simulink model "SIMWORKING"  (R2023b)
settings: Solver=VariableStepAuto  StartTime=0.0  StopTime=inf  RelTol=1e-3
undefined symbols (not defined in the file): deg, fractalcoef, IC, K, m, O, rad, s
libraries: aerolibconvert2 x7, sensorinslib x3, aerolibanimutils x3, simulink x3, aerolibnav x3, mspsensorlib x1, aerolibatmos2 x1, vrlib x1, aerolibasang x1, aerolibsim3d x1, sim3dlib x1
settings Model: Creator=kerley0  LastModifiedBy=pizza

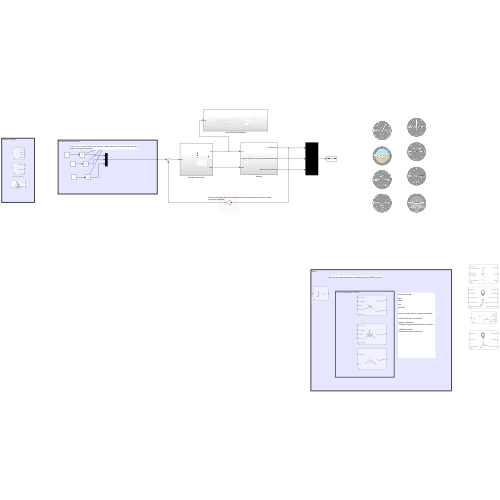
[thumbnail: Simulink's stored preview of the top-level diagram]
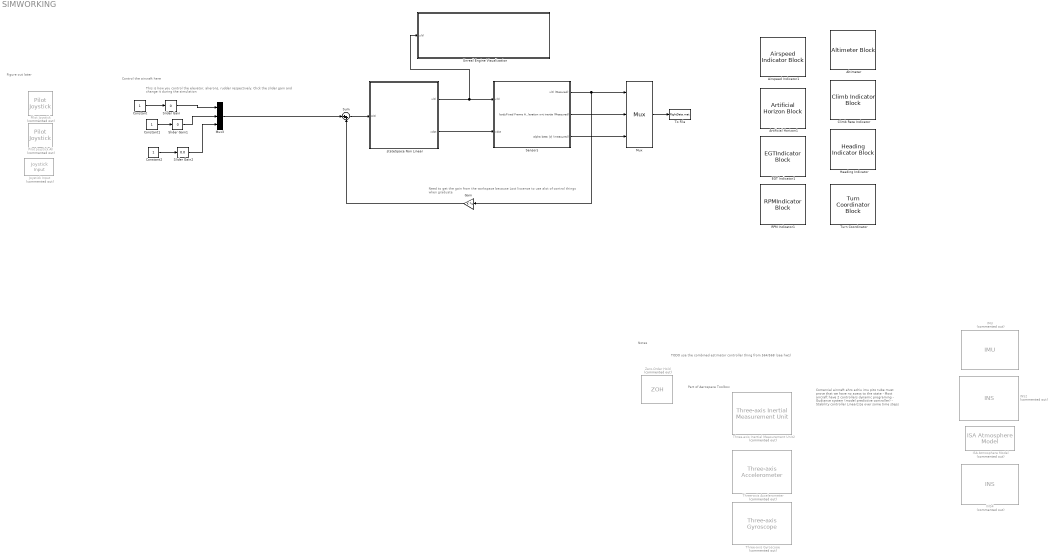
== system SIMWORKING ==
  note: Need to get the gain from the workspace because Lost liscence to use alot of control things when graduate
  note: TODO use the combined estimator controller thing from 564/568 (see hw1)
  note: Figure out later
  note: Notes
  note: Part of Aerospace Toolbox
  note: Comercial aircraft
      |
      | ahrs
      | adriu
      |
      | imu
      | pito tube
      |
      |
      | must prove that we have no acess to the state
      |
      | - Most aircraft have 2 controllers
      |
      | dynamic programing
      | - Gudiance system (model predictive controller)
      |
      | - Stability controller
      | Linearzize over some time steps
  note: Control the aircraft here
  note: This is how you control the elevator, alierons, rudder respectively. Click the slider gain and change it during the simulation
  Airspeed Indicator1 : AirspeedIndicatorBlock
  Altimeter : AltimeterBlock
  Artificial Horizon1 : ArtificialHorizonBlock
  Climb Rate Indicator : ClimbIndicatorBlock
  Constant : Constant
  Constant1 : Constant
  Constant2 : Constant
  EGT Indicator1 : EGTIndicatorBlock
  Gain : Gain  Gain=K  Multiplication=Matrix(K*u)
  Heading Indicator : HeadingIndicatorBlock
  IMU : mspsensorlib/IMU  Commented=on  DispRefFrame=NED  TemperaturePort=off  Temperature=25  MagneticFieldPort=off  MagneticFieldNED=[ 27.5550, -2.4169, -16.0849 ]  MagneticFieldENU=[ -2.4169, 27.5550, 16.0849 ]  SeedDouble=67  SimulateUsing=Interpreted execution  AccelParamsMeasurementRange=Inf  AccelParamsResolution=0  AccelParamsConstantBias=[ 0, 0, 0 ]  AccelParamsAxesMisalignment=[ 100, 0, 0; 0, 100, 0; 0, 0, 100 ]  AccelParamsNoiseDensity=[ 0, 0, 0 ]  AccelParamsBiasInstability=[ 0, 0, 0 ]  AccelParamsBiasInstabilityNumerator=fractalcoef().Numerator  AccelParamsBiasInstabilityDenominator=fractalcoef().Denominator  AccelParamsRandomWalk=[ 0, 0, 0 ]  AccelParamsNoiseType=double-sided  AccelParamsTemperatureBias=[ 0, 0, 0 ]  AccelParamsTemperatureScaleFactor=[ 0, 0, 0 ]  GyroParamsMeasurementRange=Inf  GyroParamsResolution=0  GyroParamsConstantBias=[ 0, 0, 0 ]  GyroParamsAxesMisalignment=[ 100, 0, 0; 0, 100, 0; 0, 0, 100 ]  GyroParamsAccelerationBias=[ 0, 0, 0 ]  GyroParamsNoiseDensity=[ 0, 0, 0 ]  GyroParamsBiasInstability=[ 0, 0, 0 ]  GyroParamsBiasInstabilityNumerator=fractalcoef().Numerator  GyroParamsBiasInstabilityDenominator=fractalcoef().Denominator  GyroParamsRandomWalk=[ 0, 0, 0 ]  GyroParamsNoiseType=double-sided  GyroParamsTemperatureBias=[ 0, 0, 0 ]  GyroParamsTemperatureScaleFactor=[ 0, 0, 0 ]  MagParamsMeasurementRange=Inf  MagParamsResolution=0  MagParamsConstantBias=[ 0, 0, 0 ]  MagParamsAxesMisalignment=[ 100, 0, 0; 0, 100, 0; 0, 0, 100 ]  MagParamsNoiseDensity=[ 0, 0, 0 ]  MagParamsBiasInstability=[ 0, 0, 0 ]  MagParamsBiasInstabilityNumerator=fractalcoef().Numerator  MagParamsBiasInstabilityDenominator=fractalcoef().Denominator  MagParamsRandomWalk=[ 0, 0, 0 ]  MagParamsNoiseType=double-sided  MagParamsTemperatureBias=[ 0, 0, 0 ]  MagParamsTemperatureScaleFactor=[ 0, 0, 0 ]
  INS2 : sensorinslib/INS  Commented=on  MountingLocation=[0 0 0]  RollAccuracy=0.2  PitchAccuracy=0.2  YawAccuracy=1  PositionAccuracy=1  VelocityAccuracy=0.05  UseAccelAndAngVel=on  AccelerationAccuracy=0  AngularVelocityAccuracy=0  TimeInput=off  PositionErrorFactor=[0 0 0]  SeedDouble=67  SimulateUsing=Interpreted execution
      settings: LibrarySourceBlock=uavsimlib/INS
  INS4 : sensorinslib/INS  Commented=on  MountingLocation=[0 0 0]  RollAccuracy=0.2  PitchAccuracy=0.2  YawAccuracy=1  PositionAccuracy=1  VelocityAccuracy=0.05  UseAccelAndAngVel=off  AccelerationAccuracy=0  AngularVelocityAccuracy=0  TimeInput=off  PositionErrorFactor=[0 0 0]  SeedDouble=67  SimulateUsing=Interpreted execution
      settings: LibrarySourceBlock=uavsimlib/INS
  ISA Atmosphere Model : aerolibatmos2/ISA Atmosphere Model  Commented=on  useExtended=off  action=Warning  custom=off  viscosityOut=off  g=9.80665  gamma=1.4  R=287.0531  L=0.0065  h_trop=11000  h_strat=20000  rho0=1.225  P0=101325  T0=288.15  h0=0
  Joystick Input : vrlib/Joystick Input  Commented=on  joyid=1  adjustports=on  forcefeed=off
  Mux : Mux  Inputs=3
  Mux3 : Mux  Inputs=3
  Pilot Joystick : aerolibanimutils/Pilot Joystick  Commented=on  JoystickID=Joystick1  OutputConfiguration=FourAxis  SampleTime=1/30
  Pilot Joystick All : aerolibanimutils/Pilot Joystick  Commented=on  JoystickID=Joystick1  OutputConfiguration=AllOutputs  SampleTime=1/30
      settings: LibrarySourceBlock=aerolibanimutils/Pilot Joystick All
  RPM Indicator1 : RPMIndicatorBlock
  Sensors : Subsystem
  Slider Gain : simulink/Math Operations/Slider Gain  gain=0  low=-0.4363  high=0.4363
  Slider Gain1 : simulink/Math Operations/Slider Gain  gain=0  low=-0.4363  high=0.4363
  Slider Gain2 : simulink/Math Operations/Slider Gain  gain=0.0  low=-0.6  high=0.6
  Sum : Sum  Inputs=|++
  Three-axis Accelerometer : aerolibnav/Three-axis Accelerometer  Commented=on  units=Metric (MKS)  acc=[0 0 0]  gtype=on  dtype_a=on  w_a=190  z_a=0.707  a_sf_cc=[1 0 0; 0 1 0; 0 0 1]  a_bias=[0 0 0]  a_Ts=0  a_rand=on  a_seeds=[23093 23094 23095]  a_pow=[0.001 0.001 0.001]  a_sat="[-inf  -inf  -inf  inf inf inf]"
  Three-axis Gyroscope : aerolibnav/Three-axis Gyroscope  Commented=on  dtype_g=on  w_g=190  z_g=0.707  g_sf_cc=[1 0 0; 0 1 0; 0 0 1]  g_bias=[0 0 0]  g_sen=[0 0 0]  g_Ts=0  g_rand=on  g_seeds=[23093 23094 23095]  g_pow=[0.0001 0.0001 0.0001]  g_sat="[-inf  -inf  -inf  inf inf inf]"
  Three-axis Inertial Measurement Unit2 : aerolibnav/Three-axis Inertial Measurement Unit  Commented=on  units=Metric (MKS)  imu=[0 0 0]  i_Ts=0  dtype_a=on  w_a=190  z_a=0.707  a_sf_cc=[1 0 0; 0 1 0; 0 0 1]  a_bias=[0 0 0]  a_sat="[-inf  -inf  -inf  inf inf inf]"  dtype_g=on  w_g=190  z_g=0.707  g_sf_cc=[1 0 0; 0 1 0; 0 0 1]  g_bias=[0 0 0]  g_sens=[0 0 0]  g_sat="[-inf  -inf  -inf  inf inf inf]"  i_rand=on  i_seeds=[23093 23094 23095 23096 23097 23098]  i_pow=[0.001 0.001 0.001 0.0001 0.0001 0.0001]
  To File : ToFile  Filename=flightData.mat
  Turn Coordinator : TurnCoordinatorBlock
  Unreal Engine Visualization : Subsystem
  Zero-Order Hold : ZeroOrderHold  Commented=on  SampleTime=-1
  stateSpace Non Linear : Subsystem
  wires:
  Slider Gain/1 -> Mux3/1
  Constant/1 -> Slider Gain/1
  Constant1/1 -> Slider Gain1/1
  Constant2/1 -> Slider Gain2/1
  Slider Gain2/1 -> Mux3/3
  Slider Gain1/1 -> Mux3/2
  Mux3/1 -> Sum/1
  stateSpace Non Linear/2(" xdot") -> Sensors/2(xdot)
  stateSpace Non Linear/1(x(t)) -> Sensors/1(x(t)), Unreal Engine Visualization/1(y(t))
  Sensors/3(alpha beta |V| (measured)) -> Mux/3
  Sensors/2(bodyFixed Frame Acceleration wrt inertia (Measured)) -> Mux/2
  Sensors/1(x(t) (Mesured)) -> Gain/1, Mux/1
  Mux/1 -> To File/1
  Sum/1 -> stateSpace Non Linear/1(U(t))
  Gain/1 -> Sum/2

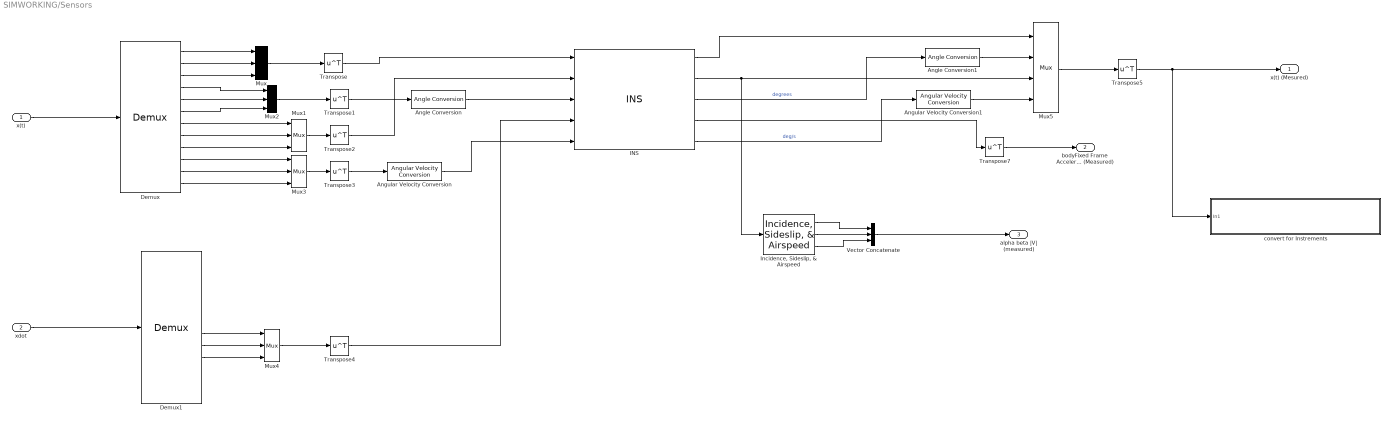
== system SIMWORKING/Sensors ==
  x(t) : Inport
  xdot : Inport  Port=2
  Angle Conversion : aerolibconvert2/Angle Conversion  IU=rad  OU=deg
  Angle Conversion1 : aerolibconvert2/Angle Conversion  IU=deg  OU=rad
  Angular Velocity Conversion : aerolibconvert2/Angular Velocity Conversion  IU=rad/s  OU=deg/s
  Angular Velocity Conversion1 : aerolibconvert2/Angular Velocity Conversion  IU=deg/s  OU=rad/s
  Demux : Demux  Outputs=12
  Demux1 : Demux  Outputs=12
  INS : sensorinslib/INS  MountingLocation=[0 0 0]  RollAccuracy=5  PitchAccuracy=5  YawAccuracy=5  PositionAccuracy=5  VelocityAccuracy=5  UseAccelAndAngVel=on  AccelerationAccuracy=1  AngularVelocityAccuracy=1  TimeInput=off  PositionErrorFactor=[0 0 0]  SeedDouble=67  SimulateUsing=Code generation
      settings: LibrarySourceBlock=mspsensorlib/INS
  "Incidence, Sideslip, & Airspeed" : aerolibasang/Incidence, Sideslip, & Airspeed
  Mux{,1..4} (5 alike) : Mux  Inputs=3
  Mux5 : Mux
  Transpose{,1..5,7} (7 alike) : Math  Operator=transpose
  Vector Concatenate : Concatenate  NumInputs=3
  convert for Instrements : Subsystem
  x(t) (Mesured) : Outport
  bodyFixed Frame Acceleration wrt inertia (Measured) : Outport  Port=2
  alpha beta |V| (measured) : Outport  Port=3
  wires:
  Transpose4/1 -> INS/4
  INS/1 -> Mux5/1
  Transpose1/1 -> Angle Conversion/1
  INS/5 -> Angular Velocity Conversion1/1  "deg/s"
  x(t)/1 -> Demux/1
  INS/3 -> Angle Conversion1/1  "degrees"
  Transpose3/1 -> Angular Velocity Conversion/1
  Demux/1 -> Mux/1
  Demux/2 -> Mux/2
  Demux/3 -> Mux/3
  Mux/1 -> Transpose/1
  Transpose/1 -> INS/1
  Demux/4 -> Mux2/1
  Demux/5 -> Mux2/2
  Demux/6 -> Mux2/3
  Mux2/1 -> Transpose1/1
  Demux/7 -> Mux1/1
  Demux/8 -> Mux1/2
  Demux/9 -> Mux1/3
  Mux1/1 -> Transpose2/1
  Transpose2/1 -> INS/2
  Demux/10 -> Mux3/1
  Demux/11 -> Mux3/2
  Demux/12 -> Mux3/3
  Mux3/1 -> Transpose3/1
  xdot/1 -> Demux1/1
  Demux1/7 -> Mux4/1
  Demux1/8 -> Mux4/2
  Demux1/9 -> Mux4/3
  Mux4/1 -> Transpose4/1
  Mux5/1 -> Transpose5/1
  Transpose5/1 -> convert for Instrements/1(In1), x(t) (Mesured)/1
  Angular Velocity Conversion/1 -> INS/5
  Angle Conversion/1 -> INS/3
  INS/2 -> "Incidence, Sideslip, & Airspeed"/1, Mux5/3
  INS/4 -> Transpose7/1
  Angular Velocity Conversion1/1 -> Mux5/4
  Angle Conversion1/1 -> Mux5/2
  "Incidence, Sideslip, & Airspeed"/1 -> Vector Concatenate/1
  "Incidence, Sideslip, & Airspeed"/2 -> Vector Concatenate/2
  "Incidence, Sideslip, & Airspeed"/3 -> Vector Concatenate/3
  Vector Concatenate/1 -> alpha beta |V| (measured)/1
  Transpose7/1 -> bodyFixed Frame Acceleration wrt inertia (Measured)/1

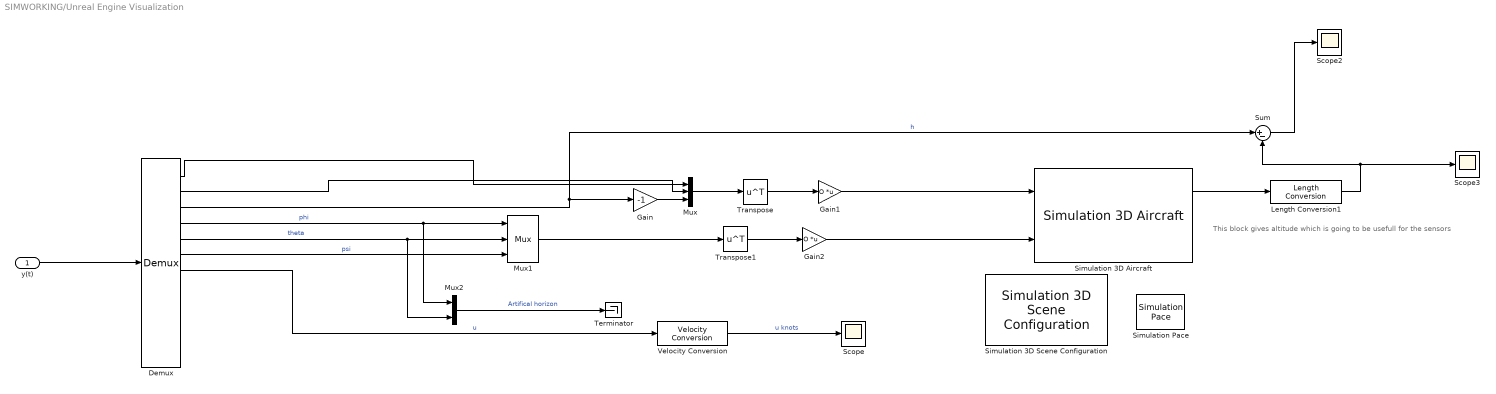
== system SIMWORKING/Unreal Engine Visualization ==
  note: This block gives altitude which is going to be usefull for the sensors
  y(t) : Inport
  Demux : Demux  Outputs=12
  Gain : Gain  Gain=-1
  Gain1 : Gain  Gain=O  Multiplication=Matrix(K*u)
  Gain2 : Gain  Gain=O  Multiplication=Matrix(K*u)
  Length Conversion1 : aerolibconvert2/Length Conversion  IU=m  OU=ft
  Mux : Mux  Inputs=3
  Mux1 : Mux  Inputs=3
  Mux2 : Mux  Inputs=2
  Scope : Scope
  Scope2 : Scope
  Scope3 : Scope
  Simulation 3D Aircraft : aerolibsim3d/Simulation 3D Aircraft  Priority=-1  Mesh=Sky Hogg  MeshPath=/MathWorksAerospaceContent/Vehicles/Aircraft/Custom/Mesh/SK_HL20.SK_HL20  MeshPathAT=/MathWorksAerospaceContent/Vehicles/Aircraft/AirTransport/Mesh/SK_AirTransport.SK_AirTransport  MeshPathGA=/MathWorksAerospaceContent/Vehicles/Aircraft/GeneralAviation/Mesh/SK_GeneralAviation.SK_GeneralAviation  AircraftColor=Red  ActorName=SimulinkVehicle1  Translation=zeros( 11, 3 )  Rotation=zeros( 11, 3 )  IsGHSensorEnabled=on  AreGHRaysVisible=off  IsOutputReshapeEnabled=off  GHRayLength=1524  GHBodyOffset=0.90  GHFrontTireRadius=0.21  GHLeftTireRadius=0.21  GHRightTireRadius=0.21  WoWSensorTolerance=0.05  LightsConfig=Automatic lights  LandingLightIntensity=300000  LandingLightConeAngle=15  CustomLeftLandingLightLocation=[0 0 0]  CustomLeftLandingLightOrientation=[0 0 0]  CustomRightLandingLightLocation=[0 0 0]  CustomRightLandingLightOrientation=[0 0 0]  TaxiLightIntensity=150000  TaxiLightConeAngle=36  CustomTaxiLightLocation=[0 0 0]  CustomTaxiLightOrientation=[0 0 0]  NavLightIntensity=500  PositionLightIntensity=500  StrobeLightIntensity=5000  WingtipStrobePeriod=1.5  WingtipStrobePulseWidth=6  TailStrobePeriod=1.5  TailStrobePulseWidth=6  BeaconLightIntensity=4000  BeaconPeriod=1.5  BeaconPulseWidth=10  SampleTime=-1  ActorType=SimulinkVehicle  ID=1  aMode=0  ActorTag=SimulinkVehicle1
  Simulation 3D Scene Configuration : sim3dlib/Simulation 3D Scene Configuration  Priority=0  ProjectFormat=Default Scenes  SceneDesc=Airport  ProjectName=C:\Program Files\MATLAB\R2023b\toolbox\shared\sim3d_projects\automotive_project_windows\UE\WindowsNoEditor\VehicleSimulation.exe  ScenePath=/Game/Maps/HwStrght  EnableOpenDRIVE=off  vehTagList={'Scene Origin';'SimulinkVehicle1'}  vehTag=SimulinkVehicle1  FreeCameraInitialTranslation=[0, 0, 0]  FreeCameraDefaultInitialTranslation=[-6, 0, 2]  FreeCameraInitialRotation=[0, 0, 0]  FreeCameraDefaultInitialRotation=[0, -15, 0]  OpVisEn=off  Ts=0.01  EnableWindow=on  EnableRemoteAccess=off  EnableWeather=off  SunAltitude=40.0  SunAzimuth=90  clouds=10  wind=1  fog=0  rain=0  EnableGeospatial=off  OriginHeight=200  OriginLatitude=40.744652  OriginLongitude=-73.988864  MapStyle=Aerial  AdditionalAssetIDs=[]  UseAdvancedSunSky=off  SolarTime=11  TimeZone=-5  Day=21  Month=9  Year=2022  UseDaylightSavingTime=on  DSTStartDay=10  DSTStartMonth=3  DSTEndDay=3  DSTEndMonth=11  DSTSwitchHour=2  sensorTag=MainCamera1  sensorId=1  sensorName=MainCamera1  mountLoc=Origin  offsetFlag=off  tmountOffset=[0, 0, 0]  rmountOffset=[0, 0, 0]  HorizontalResolution=1280  VerticalResolution=720  HorizontalFOV=60  mountPoint=[0 0 0]  mountOrientation=[0 0 0]  aMode=0  ID=1  GeoTrigger=Inactive
      settings: LibrarySourceBlock=aerolibsim3d/Simulation 3D Scene Configuration
  Simulation Pace : aerolibanimutils/Simulation Pace  SimulationPace=1  SleepMode=Auto  OutputPaceError=off  SampleTime=1/30
  Sum : Sum  Inputs=|+-
  Terminator : Terminator
  Transpose : Math  Operator=transpose
  Transpose1 : Math  Operator=transpose
  Velocity Conversion : aerolibconvert2/Velocity Conversion  IU=m/s  OU=kts
  wires:
  Gain1/1 -> Simulation 3D Aircraft/1
  Demux/6 -> Mux1/3  "psi"
  Length Conversion1/1 -> Sum/2, Scope3/1
  Demux/3 -> Gain/1, Sum/1  "h"
  Gain/1 -> Mux/3
  Transpose1/1 -> Gain2/1
  Demux/4 -> Mux2/1, Mux1/1  "phi"
  Mux2/1 -> Terminator/1  "Artifical horizon"
  Velocity Conversion/1 -> Scope/1  "u knots"
  Simulation 3D Aircraft/1 -> Length Conversion1/1
  Demux/5 -> Mux2/2, Mux1/2  "theta"
  Demux/2 -> Mux/2
  Transpose/1 -> Gain1/1
  Demux/7 -> Velocity Conversion/1  "u"
  Mux/1 -> Transpose/1
  Gain2/1 -> Simulation 3D Aircraft/2
  Mux1/1 -> Transpose1/1
  Sum/1 -> Scope2/1
  Demux/1 -> Mux/1
  y(t)/1 -> Demux/1

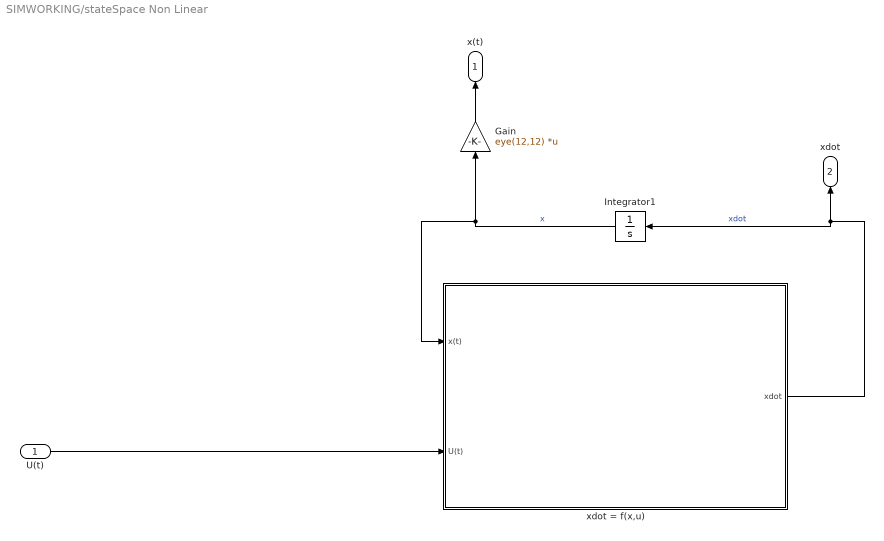
== system SIMWORKING/stateSpace Non Linear ==
  U(t) : Inport
  Gain : Gain  Gain=eye(12,12)  Multiplication=Matrix(K*u)
  Integrator1 : Integrator  InitialCondition=IC
  xdot = f(x,u) : Subsystem
  x(t) : Outport
  " xdot" : Outport  Port=2
  wires:
  xdot = f(x,u)/1(" xdot") -> " xdot"/1, Integrator1/1  "xdot"
  Integrator1/1 -> Gain/1, xdot = f(x,u)/1(x(t))  "x"
  U(t)/1 -> xdot = f(x,u)/2(U(t))
  Gain/1 -> x(t)/1

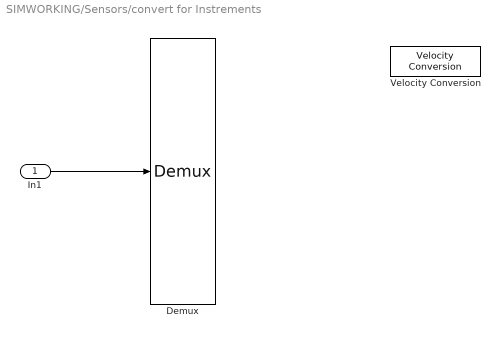
== system SIMWORKING/Sensors/convert for Instrements ==
  In1 : Inport
  Demux : Demux  Outputs=12
  Velocity Conversion : aerolibconvert2/Velocity Conversion  IU=m/s  OU=kts
  wires:
  In1/1 -> Demux/1

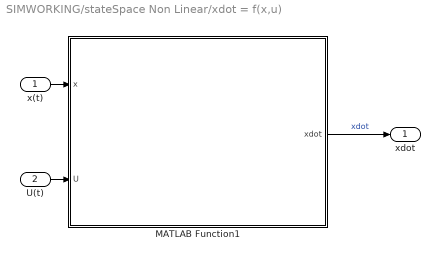
== system SIMWORKING/stateSpace Non Linear/xdot = f(x,u) ==
  x(t) : Inport
  U(t) : Inport  Port=2
  MATLAB Function1 : MATLAB Function  TreatAsAtomicUnit=on
  " xdot" : Outport
  wires:
  MATLAB Function1/1(xdot) -> " xdot"/1  "xdot"
  x(t)/1 -> MATLAB Function1/1(x)
  U(t)/1 -> MATLAB Function1/2(U)

== matlab function SIMWORKING/stateSpace Non Linear/xdot = f(x,u)/MATLAB Function1 ==
  data: x input; U input; xdot output
function xdot = dynamics(x,U)


%% Please note (This means you Aadi) 
%everything is in freedom units because thats what the flight instriments
%are compatible with
% I also cant be bothered to convert everything
%% inputs

delta_E = U(1); %elevator
delta_A = U(2); %alieron
delta_R = U(3); %rudder



%% states
X = x(1); %navigation
Y = x(2); %navigation
h = x(3); %navigation

% euler angles
phi = x(4); % about 1
theta = x(5); %about 2
psi = x(6); %bout 3

% Body frame velocities
u = x(7); %1
v = x(8); %2 
w = x(9); %3

% eWb (body frame angular velocities)
P = x(10); 
Q = x(11);
R = x(12);



%% constants

g  = 9.8; %32
W = 11787.7873; %N     %2650; %lb
m = W/g;

bw = 10.9728; %m   %36; %ft
Sw = 16.16512896; %m^2      %174; %ft^2
cBar = 1.49352; %m          %4.9; %ft
x_cm = 0; %ft




C_L_0 = 0.307; 
C_L_Alpha = 4.41; 
C_L_deltaE = 0.43;

C_DM = 0.0223;
k = 0.0554; 
C_LDM = 0;

C_M_0 = 0.04; 
C_M_Alpha = -0.613; 
C_M_deltaE = -1.122;

C_L_AlphaDot = 1.7 ; 
C_L_Q = 3.9;

C_M_AlphaDot = -7.27 ;
C_M_Q = -12.4;



C_l_beta = -0.0923; %rad^-1 421notes
C_l_deltaA = 0.005; %guess
C_l_deltaR = 1e-8; %guess
C_l_p = 0.0005; %guess
C_l_r = 0.005; %guess


C_y_beta = -0.393; %rad^-1 421notes
C_y_deltaA = 0.00005; %guess
C_y_deltaR = 0.00000005; %guess
C_y_p = 0.0005; %guess
C_y_r = 0.005; %guess

C_n_beta = 0.0587; %rad^-1 421notes
C_n_deltaA = 0.00005; %guess
C_n_deltaR = 0.00005; %guess
C_n_p = 0.000005; %guess
C_n_r = 0.000005;



rho =1.225; %kg/m^3             % 23.77e-4; %atmosisa(h)
eVbBody = [u;v;w]; %l^2 norm (euclidan) %body frame velocity in body coords
magV = norm(eVbBody);

qinf = 0.5*rho*magV^2;



alpha = atan(w/u);
beta = asin(v/magV); 
eWb = [P; Q; R]; %body frame angular velocities




%% Forces
CL = C_L_0 + C_L_Alpha *alpha + C_L_Q * Q + C_L_deltaE * delta_E;
CS = 0;
%CLstatic = C_L_0 + C_L_Alpha* alpha + C_L_E * delta_E;
CD  = C_DM + k*( CL- C_LDM) ^2; %Whatever 


L = CL*qinf*Sw; 
S = CS*qinf*Sw;
D = CD*qinf*Sw;

FxA = -D*cos(alpha)*cos(beta) -  S*cos(alpha)*sin(beta) + L *sin(alpha);
FyA = -D*sin(beta) + S*cos(alpha);
FzA = -D*sin(alpha)*cos(beta) - S*sin(alpha)*sin(beta) - L*cos(alpha);

FxP = 0;
FyP = 0;
FzP = 0; 

Fx = FxA + FxP;
Fy = FyA + FyP;
Fz = FzA + FzP;





%% Moments
Cl = C_l_beta * beta + C_l_p * P + C_l_r*R + C_l_deltaA * delta_A + C_l_deltaR*delta_R;  %rolling 
CM = C_M_0  + C_M_Alpha * alpha + C_M_Q * Q  + C_M_deltaE*delta_E;
CN = C_n_beta*beta + C_n_p * P + C_n_r*R + C_n_deltaA * delta_A + C_n_deltaR*delta_R;

lA = Cl *qinf*Sw*bw;  %rolling 
MA = CM *qinf*Sw*cBar;
NA = CN *qinf*Sw*bw;

lP = 0;  %rolling 
MP = 0; 
NP = 0;

l = lA + lP; %rolling 
M = MA + MP;
N = NA + NP;




xdot = zeros(12,1);


%% Navigation variables
p11 = [cos(psi)*cos(theta), -sin(psi)*cos(phi) + cos(psi)*sin(theta)*sin(phi), sin(psi)*sin(phi) + cos(psi)*sin(theta)*cos(phi)];
p22 = [ sin(psi)*cos(theta), cos(psi)*cos(phi) + sin(psi)*sin(theta)*sin(phi), -cos(psi)*sin(phi) + sin(psi)*sin(theta)*cos(phi) ];
p33 = [sin(theta), -cos(theta)*sin(phi), -cos(theta)*cos(phi)];

DCMb_e = [p11; p22; p33]; %% body to inertial

eVbInterial = DCMb_e * eVbBody; %body frame velocity in interial coords
xdot(1) = eVbInterial(1);
xdot(2) = eVbInterial(2);
xdot(3) = eVbInterial(3);


%% Euler angles
BodyToEuler = [1, tan(theta)*sin(phi), tan(theta)*cos(phi);
            0, cos(phi), -sin(phi);
            0, (sin(phi)/cos(theta)), (cos(phi)/cos(theta))
            ];

eulerAngleRates = BodyToEuler * eWb;

xdot(4) = eulerAngleRates(1);
xdot(5) = eulerAngleRates(2);
xdot(6) = eulerAngleRates(3);

%% velocites of body wrt interial in body frame (body fixed velocities)

udot = -Q*w + v*R - g*sin(theta) + (Fx/m);
vdot = -R*u + P*w + g*cos(theta)*sin(phi) + (Fy/m);
wdot = -P*v + Q*u + g*cos(theta)*cos(phi) + (Fz/m);

xdot(7) = udot; 
xdot(8) = vdot;
xdot(9) = wdot;



%% body fixed angular velocities represented in body frame

I11 = 1355.81; %kg m^2 %1000; %guess
I12 = 0;
I13 = 1355.81; %guess %kgm^2

I21 = 0;
I22 = 1824; %kgm^2        %1346; %slug ft^2 
I23 = 0;

I31 = I13; %kgm^2
I32 = 0;
I33 = 1016; %kgm^2        %750; %guess

Inertia = [I11 I12 I13; I21 I22 I23; I31 I32 I33];


part1 = I13*P*Q + (I22 - I33)*R*Q + l;
part2 = -I13*Q*R + (I11 - I22)*P*Q + N;
temp = (1/(I11*I33 - I13^2))*[ I33 I13; I13 I11] * [part1; part2];

Qdot = (1/I22) * ( (I33-I11) * P*R + I13*(R^2 - P^2) + M );


xdot(10) = temp(1);
xdot(11) = Qdot;
xdot(12) = temp(2);
